simulink model "q13"  (R2019a)
settings: Solver=FixedStepAuto  StartTime=0.0  StopTime=0.1  FixedStep=5e-8  RelTol=1e-3
libraries: simulink x1
settings Model: Creator=marco  LastModifiedBy=marco

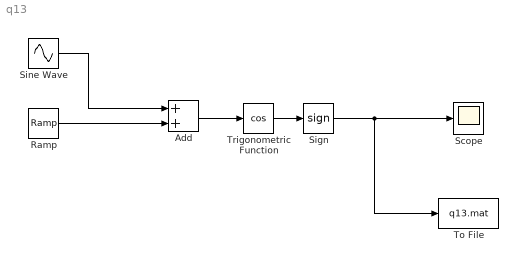
== system q13 ==
  Add : Sum
  Ramp : simulink/Sources/Ramp  slope=2*pi*(1e6)  start=0  InitialOutput=0
  Scope : Scope
  Sign : Signum
  Sine Wave : Sin  Amplitude=0.2  Frequency=2*pi*(1e4)  SampleTime=0
  To File : ToFile  Filename=q13.mat  SaveFormat=Timeseries  SampleTime=5e-8
  Trigonometric Function : Trigonometry  Operator=cos
  wires:
  Add/1 -> Trigonometric Function/1
  Sign/1 -> To File/1, Scope/1
  Trigonometric Function/1 -> Sign/1
  Ramp/1 -> Add/2
  Sine Wave/1 -> Add/1
